simulink model "func"  (R2023b)
settings: Solver=VariableStepAuto  StartTime=0.0  StopTime=10.0  RelTol=1e-3
undefined symbols (not defined in the file or in its folder): depth, x_cmd, y_cmd, yaw
libraries: ros2lib x3
settings Model: Creator=etern1ty  LastModifiedBy=etern1ty

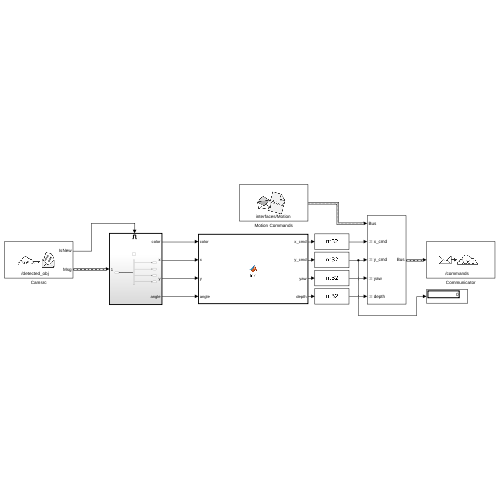
[thumbnail: Simulink's stored preview of the top-level diagram]
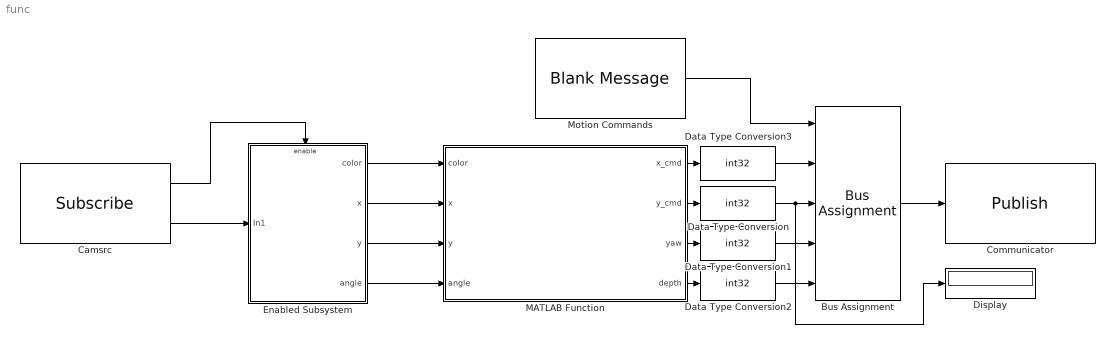
== system func ==
  Bus Assignment : BusAssignment  AssignedSignals=x_cmd,y_cmd,yaw,depth
  Camsrc : ros2lib/Subscribe  topicSource=Specify your own  topic=/detected_obj  messageType=interfaces/Detected  sampleTime=100  QOSHistory=Keep last  QOSDepth=1  QOSReliability=Reliable  QOSDurability=Volatile
  Communicator : ros2lib/Publish  topicSource=Specify your own  topic=/commands  messageType=interfaces/Motion  QOSHistory=Keep last  QOSDepth=1  QOSReliability=Reliable  QOSDurability=Volatile
  Data Type Conversion{,1..3} (4 alike) : DataTypeConversion  OutDataTypeStr=int32  SaturateOnIntegerOverflow=off  RndMeth=Floor
  Display : Display
  Enabled Subsystem : Subsystem  TreatAsAtomicUnit=on
  MATLAB Function : MATLAB Function  TreatAsAtomicUnit=on
  Motion Commands : ros2lib/Blank Message  messageClass=Message  entityType=interfaces/Motion  messageType=interfaces/Motion  SampleTime=100
  wires:
  Motion Commands/1 -> Bus Assignment/1
  Data Type Conversion/1 -> Display/1, Bus Assignment/3
  Bus Assignment/1 -> Communicator/1
  Camsrc/2 -> Enabled Subsystem/1(In1)
  Camsrc/1 -> Enabled Subsystem/Enable
  Enabled Subsystem/1(color) -> MATLAB Function/1(color)
  Enabled Subsystem/2(x) -> MATLAB Function/2(x)
  Enabled Subsystem/3(y) -> MATLAB Function/3(y)
  Enabled Subsystem/4(angle) -> MATLAB Function/4(angle)
  MATLAB Function/2(y_cmd) -> Data Type Conversion/1
  MATLAB Function/3(yaw) -> Data Type Conversion1/1
  MATLAB Function/4(depth) -> Data Type Conversion2/1
  Data Type Conversion3/1 -> Bus Assignment/2
  MATLAB Function/1(x_cmd) -> Data Type Conversion3/1
  Data Type Conversion1/1 -> Bus Assignment/4
  Data Type Conversion2/1 -> Bus Assignment/5

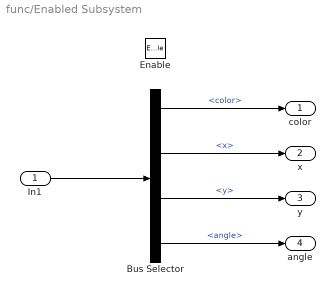
== system func/Enabled Subsystem ==
  In1 : Inport
  Enable : EnablePort
  Bus Selector : BusSelector  OutputSignals=color,x,y,angle
  color : Outport
  x : Outport  Port=2
  y : Outport  Port=3
  angle : Outport  Port=4
  wires:
  In1/1 -> Bus Selector/1
  Bus Selector/1 -> color/1  "<color>"
  Bus Selector/2 -> x/1  "<x>"
  Bus Selector/3 -> y/1  "<y>"
  Bus Selector/4 -> angle/1  "<angle>"

== matlab function func/MATLAB Function ==
  data: x_cmd output; color input; y_cmd output; x input; y input; yaw output; depth output; angle input
function [x_cmd, y_cmd, yaw, depth] = fcn(color, x, y, angle)

persistent target;

if (isempty(target))
    target = 0; % red = 0
end

x_cmd = 0;
y_cmd = 0;
yaw = 0;
depth = 0;

if (~isenum(target))

    y_cmd = 0;
    disp("Reached")

elseif (target == color)

    fprintf("Target located, moving.");
    x_cmd = x;
    yaw = int32(angle);
    depth = y;

    if ((y_cmd == 0) && (yaw == 0) && (depth == 0))
        target = target + 1;
    end

else
    fprintf("Not a target '%d'\n", int32(color));
end
